simulink model "controller_v12"  (R2022a)
settings: Solver=FixedStepDiscrete  StartTime=0.0  StopTime=inf  RelTol=1e-3
undefined symbols (not defined in the file): ctr, DiscIntNeverNeededParam, flt, IO397, mdl, rbt, rsim, som, ukf_P0_flat, ukf_prediction_time, ukf_s0, ukf_sys, ukf_use_prediction
libraries: simulink x31, slrealtimeloglib x14, slrealtimetgmanagement x5, slrealtimeseriallib x5, speedgoatlib_fpga_analog_io x4, speedgoatlib_fpga x2, speedgoatlib_fpga_dio x1, slrealtimeutilitieslib x1
(part 3 of 4)

== system controller_v12/Adaptive Controller/observer/observer/UKF ==
  r_in : Inport
  euler : Inport  Port=2
  r_dot_in : Inport  Port=3
  omega_in : Inport  Port=4
  f_cmd : Inport  Port=5
  tau_cmd_x : Inport  Port=6
  tau_cmd_y : Inport  Port=7
  To Workspace1 : ToWorkspace  VariableName=ukf_z_in  SaveFormat=Timeseries  SampleTime=-1
  To Workspace2 : ToWorkspace  VariableName=ukf_s  SaveFormat=Timeseries  SampleTime=-1
  To Workspace3 : ToWorkspace  VariableName=ukf_f_cmd  SaveFormat=Timeseries  SampleTime=-1
  To Workspace4 : ToWorkspace  VariableName=ukf_tau_cmd_x  SaveFormat=Timeseries  SampleTime=-1
  To Workspace5 : ToWorkspace  VariableName=ukf_tau_cmd_y  SaveFormat=Timeseries  SampleTime=-1
  UKF_inner : Subsystem
  euler to quat : MATLAB Function  TreatAsAtomicUnit=on
  pack measurement vector : MATLAB Function  TreatAsAtomicUnit=on
  quaternion to rotation matrix : MATLAB Function  TreatAsAtomicUnit=on
  unpack state vector : MATLAB Function  TreatAsAtomicUnit=on
  r_out : Outport
  r_dot_out : Outport  Port=2
  R_out : Outport  Port=3
  omega_out : Outport  Port=4
  wires:
  r_in/1 -> pack measurement vector/1(r)
  r_dot_in/1 -> pack measurement vector/3(r_dot)
  omega_in/1 -> pack measurement vector/4(omega)
  f_cmd/1 -> UKF_inner/2(f_cmd), To Workspace3/1
  tau_cmd_x/1 -> UKF_inner/3(tau_cmd_x), To Workspace4/1
  tau_cmd_y/1 -> To Workspace5/1, UKF_inner/4(tau_cmd_y)
  euler to quat/1(q) -> pack measurement vector/2(q)
  quaternion to rotation matrix/1(R_flat) -> R_out/1
  euler/1 -> euler to quat/1(euler_angles)
  pack measurement vector/1(z_raw) -> UKF_inner/1(z_raw), To Workspace1/1
  unpack state vector/1(r) -> r_out/1
  unpack state vector/2(q) -> quaternion to rotation matrix/1(q)
  unpack state vector/3(r_dot) -> r_dot_out/1
  unpack state vector/4(omega) -> omega_out/1
  UKF_inner/1(s_out) -> unpack state vector/1(s), To Workspace2/1

== system controller_v12/Adaptive Controller/observer/observer/UKF1 ==
  r_in : Inport
  R_in : Inport  Port=2
  f_cmd : Inport  Port=3
  tau_cmd_x : Inport  Port=4
  tau_cmd_y : Inport  Port=5
  s_prediciton_time : Inport  Port=6
  R_flat to quat : MATLAB Function  TreatAsAtomicUnit=on
  Switch : Switch  Criteria=u2 > Threshold  SaturateOnIntegerOverflow=off  InputSameDT=off
  To Workspace1 : ToWorkspace  VariableName=ukf_z_in  SaveFormat=Timeseries  SampleTime=-1
  To Workspace14 : ToWorkspace  VariableName=ukf_s_prediction_out  SaveFormat=Timeseries  SampleTime=-1
  To Workspace2 : ToWorkspace  VariableName=ukf_s  SaveFormat=Timeseries  SampleTime=-1
  To Workspace3 : ToWorkspace  VariableName=ukf_f_cmd  SaveFormat=Timeseries  SampleTime=-1
  To Workspace4 : ToWorkspace  VariableName=ukf_tau_cmd_x  SaveFormat=Timeseries  SampleTime=-1
  To Workspace5 : ToWorkspace  VariableName=ukf_tau_cmd_y  SaveFormat=Timeseries  SampleTime=-1
  UKF_inner : Subsystem
  pack measurement vector : MATLAB Function  TreatAsAtomicUnit=on
  quaternion to rotation matrix : MATLAB Function  TreatAsAtomicUnit=on
  unpack state : MATLAB Function  TreatAsAtomicUnit=on
  use prediction : Constant  Value=ukf_use_prediction
  r_out : Outport
  r_dot_out : Outport  Port=2
  R_out : Outport  Port=3
  omega_out : Outport  Port=4
  wires:
  r_in/1 -> pack measurement vector/1(r)
  f_cmd/1 -> To Workspace3/1, UKF_inner/2(f_cmd)
  tau_cmd_x/1 -> To Workspace4/1, UKF_inner/3(tau_cmd_x)
  tau_cmd_y/1 -> To Workspace5/1, UKF_inner/4(tau_cmd_y)
  R_flat to quat/1(q) -> pack measurement vector/2(q)
  quaternion to rotation matrix/1(R_flat) -> R_out/1
  pack measurement vector/1(z_raw) -> To Workspace1/1, UKF_inner/1(z_raw)
  unpack state/1(r) -> r_out/1
  unpack state/2(q) -> quaternion to rotation matrix/1(q)
  unpack state/3(r_dot) -> r_dot_out/1
  unpack state/4(omega) -> omega_out/1
  R_in/1 -> R_flat to quat/1(R_flat)
  s_prediciton_time/1 -> UKF_inner/5(s_prediction_time)
  Switch/1 -> unpack state/1(s)
  use prediction/1 -> Switch/2
  UKF_inner/2(s_out) -> To Workspace2/1, Switch/3
  UKF_inner/1(s_prediction_out) -> To Workspace14/1, Switch/1

== system controller_v12/Adaptive Controller/observer/observer/lateral observer ==
  XYZ : Inport
  derivative filter : simulink/Discrete/Transfer Fcn Lead or Lag  PoleZ=mdl.zf1  ZeroZ=1  ICPrevOutput=0.0  ICPrevInput=0.0  DoSatur=off
      settings: SourceProductBaseCode=SL
  derivative filter1 : simulink/Discrete/Transfer Fcn Lead or Lag  PoleZ=mdl.zf2  ZeroZ=1  ICPrevOutput=0.0  ICPrevInput=0.0  DoSatur=off
      settings: SourceProductBaseCode=SL
  derivative filter2 : simulink/Discrete/Transfer Fcn Lead or Lag  PoleZ=mdl.zf2  ZeroZ=1  ICPrevOutput=0.0  ICPrevInput=0.0  DoSatur=off
      settings: SourceProductBaseCode=SL
  lat_s : Gain  Gain=mdl.f1
  lat_s2 : Gain  Gain=mdl.f2
  lat_s2_ : Gain  Gain=mdl.f2
  saturation : Subsystem
  r : Outport
  r_dot : Outport  Port=2
  r_dotdot : Outport  Port=3
  wires:
  derivative filter1/1 -> derivative filter2/1
  derivative filter/1 -> lat_s/1
  XYZ/1 -> derivative filter/1, derivative filter1/1, r/1
  derivative filter2/1 -> lat_s2/1
  lat_s/1 -> r_dot/1
  lat_s2/1 -> lat_s2_/1
  lat_s2_/1 -> saturation/1(In1)
  saturation/1(Out1) -> r_dotdot/1

== system controller_v12/Adaptive Controller/observer/ICRA'23/Rotaion/filtered derivative ==
  In1 : Inport
  att_s : Gain  Gain=mdl.f1
  filtered derivative : simulink/Discrete/Transfer Fcn Lead or Lag  PoleZ=mdl.zf1  ZeroZ=1  ICPrevOutput=0.0  ICPrevInput=0.0  DoSatur=off
      settings: SourceProductBaseCode=SL
  low pass3 : DiscreteTransferFcn  Numerator=mdl.vlp.n  Denominator=mdl.vlp.d
  Out1 : Outport
  wires:
  filtered derivative/1 -> low pass3/1
  att_s/1 -> filtered derivative/1
  In1/1 -> att_s/1
  low pass3/1 -> Out1/1

== system controller_v12/Adaptive Controller/observer/ICRA'23/lateral observer/saturation ==
  In1 : Inport
  MinMax2 : MinMax  Inputs=2
  MinMax3 : MinMax  Function=max  Inputs=2
  lw1 : Constant  Value=-mdl.fd_lim
  up1 : Constant  Value=mdl.fd_lim
  Out1 : Outport
  wires:
  In1/1 -> MinMax2/2
  up1/1 -> MinMax2/1
  lw1/1 -> MinMax3/1
  MinMax2/1 -> MinMax3/2
  MinMax3/1 -> Out1/1

== system controller_v12/Adaptive Controller/observer/observer/UKF/UKF_inner ==
  z_raw : Inport
  f_cmd : Inport  Port=2
  tau_cmd_x : Inport  Port=3
  tau_cmd_y : Inport  Port=4
  Delay : Delay  DelayLength=1  InitialCondition="reshape((   diag(vertcat(   1e-4 * ones(12,1),   [0.107 * 7.2e-4; 0.107 * 7.2e-4; 0.107 * 7.2e-4],   [1.1e-21; 1.1e-21; 1e-21]   ))   )',   1,   []   )'"  SampleTime=mdl.T
  Delay1 : Delay  DelayLength=1  InitialCondition=vertcat( [0;0;0], [1;0;0;0], [0;0;0], [0;0;0], [0.981 * 7.2e-4; 0.981 * 7.2e-4; 0.981 * 7.2e-4], [5e-6;5e-6;0] )  SampleTime=mdl.T
  Delay2 : Delay  DelayLength=1  InitialCondition=zeros(13,1)  SampleTime=mdl.T
  Delay3 : Delay  DelayLength=1  InitialCondition=0  SampleTime=mdl.T
  To Workspace3 : ToWorkspace  VariableName=ukf_P_flats  SaveFormat=Timeseries  SampleTime=-1
  UKF update then predict : MATLAB Function  TreatAsAtomicUnit=on  mask{sys=ukf_sys}
  s_out : Outport
  wires:
  z_raw/1 -> UKF update then predict/1(z_raw), Delay2/1
  f_cmd/1 -> UKF update then predict/3(f_cmd)
  tau_cmd_x/1 -> UKF update then predict/4(tau_cmd_x)
  tau_cmd_y/1 -> UKF update then predict/5(tau_cmd_y)
  UKF update then predict/1(s_out) -> s_out/1, Delay1/1
  UKF update then predict/2(P_out_flat) -> Delay/1
  Delay/1 -> UKF update then predict/7(P_in_flat), To Workspace3/1
  Delay1/1 -> UKF update then predict/6(s_in)
  Delay2/1 -> UKF update then predict/2(z_raw_prev)
  UKF update then predict/3(is_init_out) -> Delay3/1
  Delay3/1 -> UKF update then predict/8(is_init_in)

== system controller_v12/Adaptive Controller/observer/observer/UKF1/UKF_inner ==
  z_raw : Inport
  f_cmd : Inport  Port=2
  tau_cmd_x : Inport  Port=3
  tau_cmd_y : Inport  Port=4
  s_prediction_time : Inport  Port=5
  Delay : Delay  DelayLength=1  InitialCondition=ukf_P0_flat  SampleTime=mdl.T
  Delay1 : Delay  DelayLength=1  InitialCondition=ukf_s0  SampleTime=mdl.T
  Delay2 : Delay  DelayLength=1  InitialCondition=[0,0,0, 1,0,0,0,0, 0,0,0, 0,0]'  SampleTime=mdl.T
  Delay3 : Delay  DelayLength=1  InitialCondition=0  SampleTime=mdl.T
  Terminator : Terminator
  To Workspace3 : ToWorkspace  VariableName=ukf_P_flats  SaveFormat=Timeseries  SampleTime=-1
  UKF update then predict : MATLAB Function  TreatAsAtomicUnit=on  mask{sys=ukf_sys}
  bee cov to SI cov : MATLAB Function  TreatAsAtomicUnit=on
  bee units to SI : MATLAB Function  TreatAsAtomicUnit=on
  bee units to SI1 : MATLAB Function  TreatAsAtomicUnit=on
  s_prediction_out : Outport
  s_out : Outport  Port=2
  wires:
  z_raw/1 -> Delay2/1, UKF update then predict/1(z_raw)
  f_cmd/1 -> UKF update then predict/3(f_cmd)
  tau_cmd_x/1 -> UKF update then predict/4(tau_cmd_x)
  tau_cmd_y/1 -> UKF update then predict/5(tau_cmd_y)
  UKF update then predict/1(s_out) -> Delay1/1, bee units to SI/1(s_bee)
  UKF update then predict/2(P_out_flat) -> Delay/1
  Delay/1 -> UKF update then predict/7(P_in_flat), bee cov to SI cov/1(P_flat_bee)
  Delay1/1 -> UKF update then predict/6(s_in)
  Delay2/1 -> UKF update then predict/2(z_raw_prev)
  UKF update then predict/3(is_init_out) -> Delay3/1
  Delay3/1 -> UKF update then predict/8(is_init_in)
  UKF update then predict/4(s_out_pre) -> Terminator/1
  bee units to SI/1(s_si) -> s_out/1
  bee cov to SI cov/1(P_flat_si) -> To Workspace3/1
  UKF update then predict/5(s_prediction_out) -> bee units to SI1/1(s_bee)
  s_prediction_time/1 -> UKF update then predict/9(s_prediction_time)
  bee units to SI1/1(s_si) -> s_prediction_out/1

== system controller_v12/Adaptive Controller/observer/observer/lateral observer/saturation ==
  In1 : Inport
  MinMax2 : MinMax  Inputs=2
  MinMax3 : MinMax  Function=max  Inputs=2
  lw1 : Constant  Value=-mdl.fd_lim
  up1 : Constant  Value=mdl.fd_lim
  Out1 : Outport
  wires:
  In1/1 -> MinMax2/2
  up1/1 -> MinMax2/1
  lw1/1 -> MinMax3/1
  MinMax2/1 -> MinMax3/2
  MinMax3/1 -> Out1/1

== matlab function controller_v12/Adaptive Controller/adaptive setpoint rd ==
  data: rd output; rd_d output; rd_dd output; rd_ddd output; rd_dddd output; time input; r input; r_d input; landing input; som_ph input; ctr parameter; som parameter; mdl parameter
function [rd,rd_d,rd_dd,rd_ddd,rd_dddd] = fcn(time, r, r_d, landing,som_ph, ctr, som, mdl)
%#codegen

rd = [ctr.setpoint.x; ctr.setpoint.y; ctr.setpoint.z];
rd_d = zeros(3,1);
rd_dd = zeros(3,1);
rd_ddd = zeros(3,1);
rd_dddd = zeros(3,1);

if time <= mdl.i_delay
    rd_z = 0;
    rd   = [ctr.setpoint.x; ctr.setpoint.y; rd_z];
end

% takeoff
if ctr.takeoff.en
    if time > mdl.i_delay && time < (mdl.i_delay+ctr.takeoff.time)
        rd_z = ctr.takeoff.height + (((ctr.setpoint.z-ctr.takeoff.height)/ctr.takeoff.time)*(time-mdl.i_delay));
        if rd_z > ctr.setpoint.z
            rd_z = ctr.setpoint.z;
        end
        rd   = [ctr.setpoint.x; ctr.setpoint.y; rd_z];
    end
end

% planned landing 
if ctr.landing.en
    if time > (mdl.rt-ctr.landing.time)
        rd_z = ctr.setpoint.z-(((ctr.setpoint.z-ctr.landing.height)/ctr.landing.time)*(time-mdl.rt+ctr.landing.time));
        if rd_z < ctr.landing.height
            rd_z = ctr.landing.height;
        end
        rd   = [ctr.setpoint.x; ctr.setpoint.y; rd_z];
    end
end

% forced landing
if landing
    rd_z = 0.02;
    rd   = [ctr.setpoint.x; ctr.setpoint.y; rd_z];
end


% somersault
if som.en
    if time > som.t_start + som.t_rise + som.t_acc + som.t_dcc + som.t_rec
        % % afterwards 
        %dt = som.t_start + som.t_rise + som.t_acc + som.t_dcc + som.t_rec - time;
        %rd = rd + dt*(r-rd);
    elseif time > som.t_start + som.t_rise + som.t_acc + som.t_dcc
        % recovery
        dt = som.t_start + som.t_rise + som.t_acc + som.t_dcc + som.t_rec - time;
        rd = rd + (dt/som.t_rec)*(r-rd);
        rd_d = rd_d + 0.5*(dt/som.t_rec)*(r_d-rd_d);
        rd(1) = min(max(rd(1),-0.25),0.25); % 25 cm envelope
        rd(2) = min(max(rd(2),-0.25),0.25); % 25 cm envelope
        rd(3) = max(rd(3),0.02); % min altitude setpoint.
    end
end


end

== matlab function controller_v12/Force//Torque to Trajectory Specs/nominal desired voltage/force to voltage (hovering) /MATLAB Function ==
  data: Vi input; Vo output; mdl parameter
function Vo = fcn(Vi,mdl)
%old script
% if max(Vi)>mdl.max_v
%     Vo = Vi * mdl.max_v/max(Vi);
%     % scale down all votages if one exceeds the max limit.
% else
%     Vo = Vi;
% end

%new change (modify max_v to a vector so each DEA has its own max)
% scale_down_ratio_vec = Vi ./ mdl.max_v_vec;
% scale_down_ratio = max(scale_down_ratio_vec);
% bool_scale_down = scale_down_ratio>1;
% 
% if bool_scale_down
%    Vo = Vi/scale_down_ratio;
% else
%    Vo = Vi; 
% end

min_v_vec = mdl.hovering_vec -150;
scale_down_ratio_vec = (Vi-min_v_vec)./(mdl.max_v_vec-min_v_vec);

scale_down_ratio = max(scale_down_ratio_vec);
bool_scale_down = scale_down_ratio>1;

if bool_scale_down
    Vo = min_v_vec + (Vi - min_v_vec)./scale_down_ratio;	
else
	  Vo = Vi; 
end


%extra layer of safety
for i=1:length(Vo)
	Vo(i) = min(Vo(i),mdl.max_v_vec(i));
end

== matlab function controller_v12/Adaptive Controller/somersault_phase ==
  data: som_phase output; time input; mdl parameter; som parameter
function som_phase  = fcn(time, mdl, som)
%#codegen

som_phase = 0;  % during a normal flight
if som.en
    if time > som.t_start + som.t_rise + som.t_acc + som.t_dcc + som.t_rec
        som_phase = 0;  % afterwards
    elseif time > som.t_start + som.t_rise + som.t_acc + som.t_dcc
        som_phase = 4;  % recovery
    elseif time > som.t_start + som.t_rise + som.t_acc
        som_phase = 3;  % rolling, second half.
    elseif time > som.t_start + som.t_rise
        som_phase = 2;  % rolling, first half.
    elseif time > som.t_start
        som_phase = 1;  % gaining altitude
    end
end

== matlab function controller_v12/Force//Torque to Trajectory Specs/nominal desired voltage/force to voltage flipping/MATLAB Function ==
  data: Vi input; Vo output; mdl parameter
function Vo = fcn(Vi,mdl)
%old script
% if max(Vi)>mdl.max_v
%     Vo = Vi * mdl.max_v/max(Vi);
%     % scale down all votages if one exceeds the max limit.
% else
%     Vo = Vi;
% end

%new change (modify max_v to a vector so each DEA has its own max)
scale_down_ratio_vec = Vi ./ mdl.max_v_vec;
scale_down_ratio = max(scale_down_ratio_vec);
bool_scale_down = scale_down_ratio>1;

if bool_scale_down
   Vo = Vi/scale_down_ratio;
else
   Vo = Vi; 
end

== matlab function controller_v12/smothing/smoothing ==
  data: time input; out_amp output; amp input; amp2 input; som parameter
function out_amp  = fcn(time,amp,amp2,som)
%#codegen

alp = 1;
if time > som.t_start + som.t_rise + som.t_acc + som.t_dcc + som.t_rec
    alp = 1;  % afterwards
elseif time > som.t_start
    alp = som.filter.alp;
end
% set en = 0 if the robot goes out of the safe envelope.
out_amp = som.filter.alp*amp + (1-som.filter.alp)*amp2;

== matlab function controller_v12/Adaptive Controller/saturation ==
  data: x_roll input; X_roll output size=1; y_pitch input; z_yaw input; Y_pitch output size=1; Z_yaw output size=1; Th input; Force output size=1; rbt parameter; ctr parameter; som_phase input; som parameter
function [X_roll, Y_pitch, Z_yaw, Force] = fcn(x_roll, y_pitch, z_yaw, Th, rbt, ctr, som_phase, som)
%#codegen

X_roll = max(min(x_roll, ctr.lim.taux), -ctr.lim.taux);
%X_roll = x_roll;
Y_pitch = max(min(y_pitch, ctr.lim.tauy), -ctr.lim.tauy);
%Y_pitch = y_pitch;
Z_yaw = max(min(z_yaw, ctr.lim.tauz), -ctr.lim.tauz);

Force = Th*rbt.m;

% F is already checked for saturation, but still needs to be converted into
% Newton

%% Roll torque management (somersault)
if som_phase == 2
    X_roll = som.roll_mag; % torque in SI
    Y_pitch = 0;  % to turn of the pitch control
elseif som_phase == 3
    X_roll = -som.roll_mag; % torque in SI
    Y_pitch = 0;  % to turn of the pitch control
end
    
%% Thrust management
% thrust is not controlled during the flipping maneuver (the output here will be overridden in the mapping).

== matlab function controller_v12/Force//Torque to Trajectory Specs/force//torque to module thrust/mapping scheme (flipping compataible) ==
  data: time input; module_f output; inputs input; rbt parameter; som parameter; mdl parameter
function module_f  = fcn(time, inputs, rbt, som, mdl)

% somersault
if som.en
    if time > som.t_start + som.t_rise + som.t_acc + som.t_dcc+som.t_rec % after recovery
        %
    elseif time > som.t_start + som.t_rise + som.t_acc + som.t_dcc % recovery
        %inputs(1) = rbt.m*(mdl.g*(som.thrust_f+0.2));
    elseif time > som.t_start + som.t_rise % rolling, first half+second half.
        % priortize the roll torque and ensure non-negative forces.
        inputs(1) = 0;
    elseif time > som.t_start
        inputs(1) = rbt.m*(mdl.g*som.thrust_f); % during the t rise.                
    end
end

% torque/thrust to unit force mapping
if rbt.til == 0
    module_f = rbt.Apinv * inputs(1:3); % original mapping
elseif rbt.til > 0
    module_f = rbt.A2inv * inputs;
else
    module_f = [0 0 0 0]';
end

% safety
if min(module_f) < 0
    module_f = module_f - min(module_f); % this ensure positive module forces
end

end

== matlab function controller_v12/Adaptive Controller/adaptive system/integrator/initial guess ==
  data: i_e input; int_e output; tor_off input; th_off input; tor_inte output; th_inte output; ctr parameter; rbt parameter; mdl parameter
function [int_e, tor_inte, th_inte] = fcn(i_e, tor_off, th_off, ctr, rbt, mdl)
%#codegen

tor_inte = zeros(3,1);
int_e    = zeros(4,1);

int_e(1) = i_e(1)+tor_off(1);
int_e(2) = i_e(2)+tor_off(2);
int_e(3) = i_e(3)+tor_off(3);
int_e(4) = i_e(4)+th_off;

tor_inte(1) = int_e(1)*ctr.gain.ati*rbt.ixx/mdl.g;
tor_inte(2) = int_e(2)*ctr.gain.ati*rbt.iyy/mdl.g;
tor_inte(3) = 0;

th_inte     = int_e(4)*ctr.gain.ali;

== matlab function controller_v12/Phantom trigger/start at one ==
  data: time input; trigger output
function trigger = fcn(time)
%#codegen
trigger = 0;
if time > 1
   trigger = 1; 
end
if time > 2
   trigger = 0; 
end

== matlab function controller_v12/Measurement manager/safety check system/envelope check ==
  data: x input; en output; y input; z input; ctr parameter
function en  = fcn(x,y,z, ctr)

if abs(x)>ctr.safety.enableZone.xmax || abs(y)>ctr.safety.enableZone.ymax || abs(z)>ctr.safety.enableZone.zmax
    en = 0;
else
    en = 1;
end

end

== matlab function controller_v12/Dynamic Sim/conditioning ==
  data: Rout output; Rin input; eu output
function [Rout, eu]  = fcn(Rin)
%#codegen
Rm = [Rin(1:3)./norm(Rin(1:3)),Rin(4:6)./norm(Rin(4:6)),Rin(7:9)./norm(Rin(7:9))];
% conditioning on orthogonality.
Rout = [Rm(:,1);Rm(:,2);Rm(:,3)];

% euler angles
euy = asin(min(max(Rm(1,3),-1),1));
eux = atan2(-Rm(2,3),Rm(3,3));
euz = atan2(-Rm(1,2),Rm(1,1));
%euz=acos(min(max(Rm(1,1)/cos(euy),-1),1));
%eux=acos(min(max(Rm(3,3)/cos(euy),-1),1));
eu = [eux;euy;euz];
% not being very careful with singularities.

== matlab function controller_v12/Force//Torque to Trajectory Specs/nominal desired voltage/map_selection ==
  data: hover_map output; time input; mdl parameter; som parameter
function hover_map  = fcn(time, mdl, som)
%#codegen

hover_map = 1;  % during a normal flight
if som.en
    if time > som.t_start + som.t_rise + som.t_acc + som.t_dcc
        hover_map = 1;  % afterwards
    elseif time > som.t_start + som.t_rise
    %elseif time > som.t_start + som.t_rise 
        hover_map = 0;  % 
    end
end

== matlab function controller_v12/Dynamic Sim/rigid body dynamics sim ==
  data: dv output double size=3; mforces input double; dR output double size=9; dw output double size=3; v input; R input; w input; rbt parameter; mdl parameter; disturbance input; rsim parameter
function [dv, dR, dw]  = fcn(mforces,v,R,w,rbt,mdl,disturbance, rsim)
%#codegen

% noiseless
% no damping
% rbt_A_temp = [rbt.A; 0.015 -0.015 0.015 -0.015];
rbt_A_temp = rbt.A2;
% inputs = rbt.A * mforces(:);
inputs = rbt_A_temp * mforces(:);
thrust = inputs(1);
% torque = [inputs(2);inputs(3);0];
torque = [inputs(2);inputs(3);inputs(4)];
%R = R(:);
%w = w(:);
dv = R(7:9)*thrust/rbt.m - [0;0;mdl.g] + disturbance(1:3);

dw = diag([rsim.rbt.ixx, rsim.rbt.iyy, rsim.rbt.izz]) \ ( (torque) - cross(w,diag([rsim.rbt.ixx, rsim.rbt.iyy, rsim.rbt.izz])*w)+ disturbance(4:6) ) ;
dR1 = R(4:6)*w(3)-R(7:9)*w(2);
dR2 = R(7:9)*w(1)-R(1:3)*w(3);
dR3 = R(1:3)*w(2)-R(4:6)*w(1);
dR = [dR1;dR2;dR3];
%dv = zeros(3,1);
%dw = zeros(3,1);
%dR = zeros(9,1);

== matlab function controller_v12/Adaptive Controller/attitude and thrust MPC controller/External Torque Observer ==
  data: time input; omega input; omega_hat output; torque_x input; torque_y input; ext_torque_hat input; omega_hat input; ext_torque_hat output; ctr parameter; rbt parameter; mdl parameter
function [omega_hat, ext_torque_hat] = fcn(time, omega, torque_x, torque_y, ext_torque_hat, omega_hat, ctr, rbt, mdl)
   
if time > mdl.i_delay
     
    omega_hat = omega_hat(:);
    ext_torque_hat = ext_torque_hat(:);
    J = diag([rbt.ixx, rbt.iyy, rbt.izz]);
    omega_cross_J_omega = cross(omega, J*omega);
    x_hat_curr = diag(ctr.torque_obs.state_scaling)*[omega_hat(:); ext_torque_hat(:)];
    u = diag(ctr.torque_obs.input_scaling)*[torque_x - omega_cross_J_omega(1); torque_y - omega_cross_J_omega(2)];
    y = diag(ctr.torque_obs.meas_scaling)*omega(1:2); 
    x_hat_pred = ctr.torque_obs.A*x_hat_curr + ctr.torque_obs.B(:, 1:2)*u; 
    x_hat_next = diag(ctr.torque_obs.out_scaling)*(x_hat_pred + ctr.torque_obs.L*(y - ctr.torque_obs.C*x_hat_pred));
    omega_hat = x_hat_next(1:2,1);
    ext_torque_hat = x_hat_next(3:4,1);
end

end

== matlab function controller_v12/Measurement manager/safety check system/voltage check ==
  data: voltage input; en output; ctr parameter
function en  = fcn(voltage, ctr)

if sum(voltage>ctr.safety.volt) > 0
    en = 0;
else
    en = 1;
end

end

== matlab function controller_v12/Measurement manager/envelope//voltage check ==
  data: x input; keep_flying output size=1; y input; z input; ctr parameter
function keep_flying  = fcn(x,y,z,ctr)

if abs(x)>ctr.safety.land.xmax || abs(y)>ctr.safety.land.ymax || abs(z)>ctr.safety.land.zmax
    keep_flying = 0;
% elseif voltage(1) > ctr.safety.land.volt
%     keep_flying = 0;    
else
    keep_flying = 1;
end

end

== matlab function controller_v12/Measurement manager/MATLAB Function ==
  data: keep_flying input; landing_in input; landing_out output size=1; cum_in input; cum_out output size=1; ctr parameter; mdl parameter
function [landing_out, cum_out] = fcn(keep_flying, landing_in, cum_in, ctr, mdl)

if keep_flying == 0
    cum_out = cum_in + mdl.T;
else
    cum_out = 0;
end

if cum_out > ctr.safety.land.T || landing_in == 1
    landing_out = 1;
else 
    landing_out = 0;
end

end

== matlab function controller_v12/Measurement manager/voltage check ==
  data: voltage input; keep_flying output size=1; ctr parameter
function keep_flying  = fcn(voltage, ctr)

% if voltage(1)>ctr.safety.land.volt || voltage(2)>ctr.safety.land.volt || voltage(3)>ctr.safety.land.volt || voltage(4)>ctr.safety.land.volt

if sum(voltage>ctr.safety.land.volt)>0
    keep_flying = 0;
else
    keep_flying = 1;
end

end

== matlab function controller_v12/Measurement manager/safety check system/MATLAB Function ==
  data: keep_flying input; en_in input; en_out output size=1; cum_in input; cum_out output size=1; ctr parameter; mdl parameter
function [en_out, cum_out] = fcn(keep_flying, en_in, cum_in, ctr, mdl)

if keep_flying == 0
    cum_out = cum_in + mdl.T;
else
    cum_out = 0;
end

if cum_out > ctr.safety.T || en_in == 0
    en_out = 0;
else 
    en_out = 1;
end

end

== matlab function controller_v12/MATLAB Function ==
  data: u input; y output
function y = fcn(u)

y = u;

== matlab function controller_v12/Adaptive Controller/attitude and thrust MPC controller/PD Atttiude Controller ==
  data: time input; cmd_B_torque output; R input; Omega input; Rd input; Omegad input; tau_ext input; ctr parameter; rbt parameter; mdl parameter; att_e output
function [cmd_B_torque, att_e]   = fcn(time, R, Omega, Rd, Omegad, tau_ext, ctr, rbt, mdl)
%#codegen
% r: curr pos
% r_dot: curr vel
% R: current attitude
% Omega: current body rates
% rd : des pos
% rd_d: des vel
% Rd: desired attitude (rotation matrix)
% Omegad: desired angular velocity


% current attitude
R = get_rotation_matrix(R);     % transform vector in rotation matrix
Omega = Omega(:);
Omegad = Omegad(:);

% desired attitude & angvel
Rd = get_rotation_matrix(Rd);

B_ypr_curr = rotm2eul(R);
B_ypr_des = rotm2eul(Rd);

B_ypr_dot_des = get_euler_derivatives(B_ypr_des, Omegad);
B_ypr_dot_curr = get_euler_derivatives(B_ypr_curr, Omega);
B_ypr_e_dot = (B_ypr_dot_curr - B_ypr_dot_des);
B_rpy_e_dot = [B_ypr_e_dot(3); B_ypr_e_dot(2); B_ypr_e_dot(1)];
disp(B_rpy_e_dot)
disp(Omega - Omegad)

B_ypr_e = B_ypr_curr - B_ypr_des;
B_rpy_e = [B_ypr_e(3); B_ypr_e(2); B_ypr_e(1)];
M = diag(ctr.att_pid_e)*B_rpy_e + diag(ctr.att_pid_e_dot)*B_rpy_e_dot + [tau_ext(1); tau_ext(2); 0.0];

%att_e = eR'*eR; % squared norm of the error
att_e = B_rpy_e(:);
cmd_B_torque = M(:);
end

function R = get_rotation_matrix(R)
    R11 = R(1);
    R12 = R(2);
    R13 = R(3);
    R21 = R(4);
    R22 = R(5);
    R23 = R(6);
    R31 = R(7);
    R32 = R(8);
    R33 = R(9);
    R1 = [R11; R21; R31];     % unit (column) vector
    R2 = [R12; R22; R32];
    R3 = [R13; R23; R33];
    R = [R1, R2, R3];
end

function [B_ypr_dot] = get_euler_derivatives(B_ypr, B_omega)
% https://www.astro.rug.nl/software/kapteyn-beta/_downloads/attitude.pdf
sy = sin(B_ypr(1));
cy = cos(B_ypr(1));
sp = sin(B_ypr(2));
cp = cos(B_ypr(2));
E_zyx = [[0; 0; 1], [-sy; cy; 0.0], [cy*cp; sy*cp; -sp]];
B_ypr_dot = E_zyx\B_omega;

end

== matlab function controller_v12/Adaptive Controller/attitude and thrust MPC controller/Pakpong;s atttiude ==
  data: time input; R input; Omega input; Rd input; Omegad input; cmd_B_acc_z input; cmd_B_torque output; ctr parameter; rbt parameter; mdl parameter; att_e output
function [cmd_B_torque, att_e]   = fcn(time, R, Omega, Rd, Omegad, cmd_B_acc_z, ctr, rbt, mdl)
%#codegen

%% init
R11 = R(1);
R12 = R(2);
R13 = R(3);
R21 = R(4);
R22 = R(5);
R23 = R(6);
R31 = R(7);
R32 = R(8);
R33 = R(9);
R1 = [R11; R21; R31];     % unit (column) vector
R2 = [R12; R22; R32];
R3 = [R13; R23; R33];
R = [R1, R2, R3];
wx = Omega(1);
wy = Omega(2);
wz = Omega(3);

e3 = [0; 0; 1];
rd_dd = get_rotation_matrix(Rd)*e3*cmd_B_acc_z;

torque_x = ...
- ctr.gain.at3*( mdl.g*wx) - ...
ctr.gain.at2*( dot(R2,rd_dd) );
torque_x = torque_x*rbt.ixx/mdl.g;

torque_y = ...
- ctr.gain.at3*( mdl.g*wy) - ...
ctr.gain.at2*( dot(R1,-rd_dd) );
torque_y = torque_y*rbt.iyy/mdl.g;

torque_z = 0;           % no yaw control

att_e = -[-dot(R2,rd_dd);dot(R1,rd_dd);0];

cmd_B_torque = [torque_x; torque_y; torque_z];

end

function R = get_rotation_matrix(R)
    R11 = R(1);
    R12 = R(2);
    R13 = R(3);
    R21 = R(4);
    R22 = R(5);
    R23 = R(6);
    R31 = R(7);
    R32 = R(8);
    R33 = R(9);
    R1 = [R11; R21; R31];     % unit (column) vector
    R2 = [R12; R22; R32];
    R3 = [R13; R23; R33];
    R = [R1, R2, R3];

end

== matlab function controller_v12/Adaptive Controller/attitude and thrust MPC controller2/Geometric Attitude Controller ==
  data: time input; torque_x output; R input; Omega input; Rd input; Omegad input; ctr parameter; rbt parameter; torque_y output; torque_z output; mdl parameter; att_e output
function [torque_x, torque_y, torque_z, att_e]   = fcn(time, R, Omega, Rd, Omegad, ctr, rbt, mdl)
%#codegen
% r: curr pos
% r_dot: curr vel
% R: current attitude
% Omega: current body rates
% rd : des pos
% rd_d: des vel
% Rd: desired attitude (rotation matrix)
% Omegad: desired angular velocity


% current attitude
R = get_rotation_matrix(R);     % transform vector in rotation matrix
Omega = Omega(:);

% desired attitude & angvel
Rd = get_rotation_matrix(Rd);
Omegad = Omegad(:);
% Omegad      = [0; 0; 0]; % vee(Rd.'*Rd_1dot);
Omegad_1dot = [0; 0; 0]; % vee(Rd.'*Rd_2dot - hat(Omegad)*hat(Omegad));

% inertia matrix
J = diag([ctr.lee.ixx, ctr.lee.iyy, ctr.lee.izz]);

% attitude and angular velocity errors
eR     = (1/2)*vee(Rd.'*R - R.'*Rd);
eOmega = Omega - R.'*Rd*Omegad;

% desired torque
M = -ctr.lee.kR*eR - ctr.lee.kOmega*eOmega + cross(Omega, J*Omega) ...
  - J*(hat(Omega)*R.'*Rd*Omegad - R.'*Rd*Omegad_1dot);

%att_e = eR'*eR; % squared norm of the error
att_e = eR;

torque_x = M(1);
torque_y = M(2);
torque_z = M(3);

end

function vec = vee(ss)
% function vec = vee(skewsymmetric)
%   The vee function maps a skew-symmetric 
%   matrix to a vector

% https://github.com/justinthomas/MATLAB-tools/blob/master/vee.m

if isa(ss,'sym')
    ss = expand(simplify(ss));
end

switch numel(ss)
    
    case 4
        
        if ~isequal(ss(1,2), -ss(2,1))
            %warning('The provided matrix is not skew symmetric')
        end
        
        vec = ss(1,2);

    case 9

        if ~isequal(ss(3,2),-ss(2,3)) || ~isequal(ss(1,3),-ss(3,1)) || ~isequal(ss(2,1),-ss(1,2))
            %warning('The provided matrix is not skew symmetric.')
            %print(ss)
        end

        vec = [ss(3,2); ss(1,3); ss(2,1)];
end

if isa(ss,'sym')
    vec = simplify(vec);
end

end

function ss = hat(vec)
% function ss = hat(vec)
%   The hat function maps a vector in R^3 (or R^1) to its
%   skew symmetric matrix in R^(3x3) (or R^(2x2))

% https://github.com/justinthomas/MATLAB-tools/blob/master/hat.m

switch length(vec)
    
    case 3
        ss = [...
            0, -vec(3), vec(2);...
            vec(3), 0, -vec(1);...
            -vec(2), vec(1), 0];
        
    case 1
        ss = [...
            0, vec; ...
            -vec, 0];
end

end

function R = get_rotation_matrix(R)
    R11 = R(1);
    R12 = R(2);
    R13 = R(3);
    R21 = R(4);
    R22 = R(5);
    R23 = R(6);
    R31 = R(7);
    R32 = R(8);
    R33 = R(9);
    R1 = [R11; R21; R31];     % unit (column) vector
    R2 = [R12; R22; R32];
    R3 = [R13; R23; R33];
    R = [R1, R2, R3];

end

== matlab function controller_v12/Adaptive Controller/attitude and thrust MPC controller2/MATLAB Function ==
  data: u input; y output
function y = fcn(u)

y = u;

== matlab function controller_v12/Adaptive Controller/attitude and thrust MPC controller/Geometric Attitude Controller ==
  data: time input; cmd_B_torque output; R input; Omega input; Rd input; Omegad input; tau_ext input; ctr parameter; rbt parameter; mdl parameter; att_e output
function [cmd_B_torque, att_e]   = fcn(time, R, Omega, Rd, Omegad, tau_ext, ctr, rbt, mdl)
%#codegen
% r: curr pos
% r_dot: curr vel
% R: current attitude
% Omega: current body rates
% rd : des pos
% rd_d: des vel
% Rd: desired attitude (rotation matrix)
% Omegad: desired angular velocity


% current attitude
R = get_rotation_matrix(R);     % transform vector in rotation matrix
Omega = Omega(:);
Omegad = Omegad(:);

% desired attitude & angvel
Rd = get_rotation_matrix(Rd);
% inertial frame 3-axis



% thrust magnitude control, eq 19
%A = -ctr.lee.pos.kx*ex - ctr.lee.pos.kv*ev - rbt.m*mdl.g*e3; % + P.mass*xd_2dot;
%cmd_B_acc_z = dot(-A, R*e3)/rbt.m;

Rd = get_desired_attitude_x_axis(Rd, R);
%Rd = get_desired_attitude_y_axis(Rd, R);

% inertia matrix
J = diag([ctr.lee.ixx, ctr.lee.iyy, ctr.lee.izz]);

% attitude and angular velocity errors
eR     = (1/2)*vee(Rd.'*R - R.'*Rd);
eOmega = Omega - R.'*Rd*Omegad;
% desired torque
M = -ctr.lee.kR*eR - ctr.lee.kOmega*eOmega + cross(Omega, J*Omega)...
    - J*(hat(Omega)*R.'*Rd*Omegad) ...
    - ctr.torque_obs.factor.*[tau_ext(1); tau_ext(2); 0.0]; % ...
  % - J*(- R.'*Rd*Omegad_1dot);
  % - J*(hat(Omega)*R.'*Rd*Omegad) ...

%att_e = eR'*eR; % squared norm of the error
att_e = eR;
cmd_B_torque = M(:);
end

function vec = vee(ss)
% function vec = vee(skewsymmetric)
%   The vee function maps a skew-symmetric 
%   matrix to a vector

% https://github.com/justinthomas/MATLAB-tools/blob/master/vee.m

if isa(ss,'sym')
    ss = expand(simplify(ss));
end

switch numel(ss)
    
    case 4
        
        if ~isequal(ss(1,2), -ss(2,1))
            disp('The provided matrix is not skew symmetric')
        end
        
        vec = ss(1,2);

    case 9

        if ~isequal(ss(3,2),-ss(2,3)) || ~isequal(ss(1,3),-ss(3,1)) || ~isequal(ss(2,1),-ss(1,2))
            disp('The provided matrix is not skew symmetric.')
            %print(ss)
        end

        vec = [ss(3,2); ss(1,3); ss(2,1)];
end

if isa(ss,'sym')
    vec = simplify(vec);
end

end

function ss = hat(vec)
% function ss = hat(vec)
%   The hat function maps a vector in R^3 (or R^1) to its
%   skew symmetric matrix in R^(3x3) (or R^(2x2))

% https://github.com/justinthomas/MATLAB-tools/blob/master/hat.m

switch length(vec)
    
    case 3
        ss = [...
            0, -vec(3), vec(2);...
            vec(3), 0, -vec(1);...
            -vec(2), vec(1), 0];
        
    case 1
        ss = [...
            0, vec; ...
            -vec, 0];
end

end

function R = get_rotation_matrix(R)
    R11 = R(1);
    R12 = R(2);
    R13 = R(3);
    R21 = R(4);
    R22 = R(5);
    R23 = R(6);
    R31 = R(7);
    R32 = R(8);
    R33 = R(9);
    R1 = [R11; R21; R31];     % unit (column) vector
    R2 = [R12; R22; R32];
    R3 = [R13; R23; R33];
    R = [R1, R2, R3];

end

function Omegad = get_desired_body_velocity()

% time derivatives of body axes -- arXiv:1003.2005v3, Appendix F
A_1dot   = -ctr.lee.pos.kx*ev; %- ctr.lee.pos.kv*ea + ctr.lee.pos.mass*xd_3dot;
b3c_1dot = -A_1dot/norm(A) + (dot(A,A_1dot)/norm(A)^3)*A;
C_1dot   = cross(b3c_1dot, b1d) + cross(b3c, b1d_1dot);
b2c_1dot = C/norm(C) - (dot(C,C_1dot)/norm(C)^3)*C;
% b2c_1dot = -1*b2c_1dot;
b1c_1dot = cross(b2c_1dot, b3c) + cross(b2c, b3c_1dot);

% Extract calculated angular velocities and their time-derivatives
Rd_1dot     = [b1c_1dot b2c_1dot b3c_1dot];
Omegad      = vee(Rd_tmp.'*Rd_1dot);

% Omegad      = [0; 0; 0]; % vee(Rd.'*Rd_1dot);
Omegad_1dot = [0; 0; 0]; % vee(Rd.'*Rd_2dot - hat(Omegad)*hat(Omegad));

end

function Rd = get_desired_attitude_x_axis(Rd, R)

    e3 = [0;0;1];
    % normalized feedback function, eq 23
    b3c = Rd*e3;
    
    % Desired x axis -- current x axis
    b1d = R(:, 1);
    
    % Construct b1c, eq 38
    C = cross(b3c, b1d); % arXiv:1003.2005v3, eq ~97
    b1c = -(1/norm(C))*cross(b3c, C);
    
    b2c = C/norm(C);
    
    % computed attitude, eq 22
    Rd = [b1c b2c b3c];

end


function Rd = get_desired_attitude_y_axis(Rd, R)

    e3 = [0;0;1];
    % normalized feedback function, eq 23
    b3c = Rd*e3;
    
    % Desired y axis -- current x axis
    b2d = R(:, 2);
    
    % Construct b2c, eq 38
    C = cross(b3c, b2d); % arXiv:1003.2005v3, eq ~97
    b2c = -(1/norm(C))*cross(b3c, C);
    
    b1c = C/norm(C);
    
    % computed attitude, eq 22
    Rd = [b1c b2c b3c];

end

== matlab function controller_v12/Adaptive Controller/attitude and thrust MPC controller/Geometric Controller ==
  data: time input; r input; Rd output; r_dot input; r_dotdot input; R input; Omega input; rd input; rd_d input; rd_dd input; rd_ddd input; rd_dddd input; int_e input; ctr parameter; rbt parameter; Omegad output; cmd_B_acc_z output; mdl parameter; alt_e output; rd_rtmpc output
function [Rd, Omegad, cmd_B_acc_z, alt_e, rd_rtmpc]   = fcn(time, r, r_dot, r_dotdot, R, Omega, rd,rd_d,rd_dd,rd_ddd,rd_dddd, int_e, ctr, rbt, mdl)
    %#codegen
    % r: curr pos
    % r_dot: curr vel
    % R: current attitude
    % Omega: current body rates
    % rd : des pos
    % rd_d: des vel
    %% Out: 
    % cmd_B_thrust_z is thrust force on z axis in body (B) frame [N]
    
    % Ensure signals have expected shape
    R11 = R(1);
    R12 = R(2);
    R13 = R(3);
    R21 = R(4);
    R22 = R(5);
    R23 = R(6);
    R31 = R(7);
    R32 = R(8);
    R33 = R(9);
    R1 = [R11; R21; R31];     % unit (column) vector
    R2 = [R12; R22; R32];
    R3 = [R13; R23; R33];
    R = [R1, R2, R3];

    r = r(:);           % position
    r_dot = r_dot(:);   % velocity 

    rd = rd(:);         % desired position
    rd_d = rd_d(:);     % desired velocity

    rd_rtmpc = [rd; rd_d];

    
    % From https://github.com/plusk01/se3quad/blob/master/matlab/controller.m
    % calculate errors, eq 17-18
    ex = r - rd;
    ev = r_dot - rd_d;
    %ea = v_1dot - xd_2dot;
    %ej = v_2dot - xd_3dot;
    
    % inertial frame 3-axis
    e3 = [0;0;1];
    
    % thrust magnitude control, eq 19
    A = -ctr.lee.pos.kx*ex - ctr.lee.pos.kv*ev - rbt.m*mdl.g*e3; % + P.mass*xd_2dot;
    cmd_B_acc_z = dot(-A, R*e3)/rbt.m;
    
    % normalized feedback function, eq 23
    b3c = -A/norm(A);

    % Desired x axis -- current x axis
    b1d = R(:, 1);
    % Desired angular velocity of this axis - zero?
    b1d_1dot = [0; 0; 0];
    
    % Construct b1c, eq 38
    C = cross(b3c, b1d); % arXiv:1003.2005v3, eq ~97
    b1c = -(1/norm(C))*cross(b3c, C);
    
    b2c = C/norm(C);
    
    % computed attitude, eq 22
    Rd_tmp = [b1c b2c b3c];

    % time derivatives of body axes -- arXiv:1003.2005v3, Appendix F
    A_1dot   = -ctr.lee.pos.kx*ev; %- ctr.lee.pos.kv*ea + ctr.lee.pos.mass*xd_3dot;
    b3c_1dot = -A_1dot/norm(A) + (dot(A,A_1dot)/norm(A)^3)*A;
    C_1dot   = cross(b3c_1dot, b1d) + cross(b3c, b1d_1dot);
    b2c_1dot = C/norm(C) - (dot(C,C_1dot)/norm(C)^3)*C;
    % b2c_1dot = -1*b2c_1dot;
    b1c_1dot = cross(b2c_1dot, b3c) + cross(b2c, b3c_1dot);
    
    % Extract calculated angular velocities and their time-derivatives
    Rd_1dot     = [b1c_1dot b2c_1dot b3c_1dot];
    Omegad      = vee(Rd_tmp.'*Rd_1dot);

    % Desired angular velocity
    % Omegad = [0.0, 0.0, 0.0]; % TODO

    % Altitude error
    alt_e = r(3) - rd(3); 

    % Generate output. 
    Rd_tmp = Rd_tmp'; % this is needed to respect existing convention that rot. matrices are passed
          % around as vectors, created by concatenating the rows of the
          % matrix (and Rd(:) will created a vector by concatentatig the columns of Rd)
    Rd = Rd_tmp(:);
end

function [B_thrust] = compensate_thrust(cmd_B_acc_z, B_ypr, mass, g)
    B_thrust_z = mass * (cmd_B_acc_z+g)/cos(B_ypr(3))/cos(B_ypr(2));
    B_thrust = [0.0; 0.0; B_thrust_z];
end

function [B_roll, B_pitch] = compensate_attitude(B_thrust, lin_B_roll, lin_B_pitch, mass, g)
    B_acc_z = (B_thrust(3))/mass;
    B_roll = lin_B_roll*(g/B_acc_z);
    B_pitch = lin_B_pitch*(g/B_acc_z);
end

function [R] = get_B_R_yaw_I(yaw)
    R = [cos(yaw), sin(yaw); -sin(yaw), cos(yaw)];
end

function vec = vee(ss)
% function vec = vee(skewsymmetric)
%   The vee function maps a skew-symmetric 
%   matrix to a vector

% https://github.com/justinthomas/MATLAB-tools/blob/master/vee.m

if isa(ss,'sym')
    ss = expand(simplify(ss));
end

switch numel(ss)
    
    case 4
        
        if ~isequal(ss(1,2), -ss(2,1))
            %warning('The provided matrix is not skew symmetric')
        end
        
        vec = ss(1,2);

    case 9

        if ~isequal(ss(3,2),-ss(2,3)) || ~isequal(ss(1,3),-ss(3,1)) || ~isequal(ss(2,1),-ss(1,2))
            %warning('The provided matrix is not skew symmetric.')
            %print(ss)
        end

        vec = [ss(3,2); ss(1,3); ss(2,1)];
end

if isa(ss,'sym')
    vec = simplify(vec);
end

end

== matlab function controller_v12/Adaptive Controller/attitude and thrust MPC controller/RTMPC Trajectory Tracking ==
  data: time input; r input; Rd output; r_dot input; r_dotdot input; R input size=9; Omega input; rd input; rd_d input; rd_dd input; rd_ddd input; rd_dddd input; att_cmd input; int_e input; ctr parameter; rbt parameter; Omegad output; cmd_B_acc_z output size=1; mdl parameter; alt_e output; rd_rtmpc output; new_att_cmd output
function [Rd, Omegad, cmd_B_acc_z, alt_e, rd_rtmpc, new_att_cmd]   = fcn(time, r, r_dot, r_dotdot, R, Omega, rd,rd_d,rd_dd,rd_ddd,rd_dddd, att_cmd, int_e, ctr, rbt, mdl)
    %#codegen
    % r: curr pos
    % r_dot: curr vel
    % R: current attitude
    % Omega: current body rates
    % rd : des pos
    % rd_d: des vel
    cmd_B_acc_z = 0;
    %% Out: 
    % cmd_B_thrust_z is thrust force on z axis in body (B) frame [N]
    
    % Ensure signals have expected shape
    R11 = R(1);
    R12 = R(2);
    R13 = R(3);
    R21 = R(4);
    R22 = R(5);
    R23 = R(6);
    R31 = R(7);
    R32 = R(8);
    R33 = R(9);
    R1 = [R11; R21; R31];     % unit (column) vector
    R2 = [R12; R22; R32];
    R3 = [R13; R23; R33];
    R = [R1, R2, R3];

    r = r(:);           % position
    r_dot = r_dot(:);   % velocity 

    rd = rd(:);         % desired position
    rd_d = rd_d(:);     % desired velocity

    new_att_cmd = zeros(2,1);
    Omegad = [0.0; 0.0; 0.0];
    
    % Compute current attitude as euler angles (:( )
    B_ypr = rotm2eul(R);
    B_est_roll = B_ypr(3);
    B_est_pitch = B_ypr(2);
    B_est_yaw = B_ypr(1);

    % Conver attitude in yaw-invariant frame. 
    B_R_yaw_I = get_B_R_yaw_I(B_est_yaw);
    I_rp = B_R_yaw_I'*[B_est_roll; B_est_pitch];

    % Generate reference % (currently only circle is supported)
    x_ref = traj_planner(time, ctr.rtmpc.ref_len, ctr.rtmpc.traj, ctr);

    % Set current state
    x = [r - ctr.rtmpc.r_origin; r_dot; I_rp(1); I_rp(2);];

    if ctr.mode == 0
        % NN RTMPC controller

        % Apply state and reference scaling
        x = [x; att_cmd(1); att_cmd(2)];
        x_scaled = ctr.rtmpc.in_scaling.*x;
        x_ref_scaled = repmat(ctr.rtmpc.in_scaling(1:6), ctr.rtmpc.ref_len, 1).*x_ref;
        
        x_in = [x_scaled; x_ref_scaled];
        x_in = x_in(:); % column vector

        % 10.0 and 12.0 are some scalings applied to the NN to
        % ensure that its input/ouput is in [-1, 1]. 
        % For the rtmpc expert we do not have this care -- but we scale
        % things to ensure that input/outpurs are not too large numbers (e.g., <+-100)
        u_next = 10.0*rtmpcnn(x_in/10.0, ctr.rtmpc.nnparam);

        % Apply rtmpc scaling: 
        u_next = u_next.*ctr.rtmpc.out_scaling;

        % integrated new att cmd
        new_att_cmd = zeros(2,1);
        new_att_cmd(:, 1) = mdl.T*u_next(1:2) + att_cmd;

        % Approach 2: rotate in B after.
        Iy_rp_des_dot = [u_next(1); u_next(2)];
        Iy_rp_des = [new_att_cmd(1); new_att_cmd(2)];
        % compute angular velocity in yaw-aligned frame
        Iy_ypr_des = [0.0; Iy_rp_des(2); Iy_rp_des(1)];
        Iy_ypr_des_dot = [0.0; Iy_rp_des_dot(2); Iy_rp_des_dot(1)];
        Iy_Omegad = get_body_ang_vel(Iy_ypr_des, Iy_ypr_des_dot);
        B_R_yaw_I = get_B_R_yaw_I(B_est_yaw);
        B_Omegad_12 = B_R_yaw_I*Iy_Omegad(1:2);
        Omegad = [B_Omegad_12(1); B_Omegad_12(2); 0.0];
        u_next(1:2) = new_att_cmd;

    elseif ctr.mode == 1
        
        % Set reference 
        %x_ref = [rd; rd_d; 0.0; 0.0]; % no attitude feed-forward at the moment. 
        %mpc.set_reference_trajectory(x_ref);
    
        % Compute new linearized commands
        x = [r; r_dot; I_rp(1); I_rp(2)];

        x_scaled = x.*ctr.lqrv2.in_scaling;
        x_ref_scaled = [x_ref(1:6); 0.0; 0.0;].*ctr.lqrv2.in_scaling;
        u_next = -ctr.lqrv2.K*(x_scaled - x_ref_scaled);
        u_next = u_next.*ctr.lqrv2.out_scaling;
        Omegad = zeros(3, 1);

    elseif ctr.mode == 2
        x = [x; att_cmd(1); att_cmd(2)];
        ctr.lqr.in_scaling = [10; 10; 10; 10; 10; 10; 1; 1; 1; 1];
        x_scaled = x.*ctr.lqr.in_scaling;
        x_ref_scaled = [x_ref(1:6); 0.0; 0.0; 0.0; 0.0;].*ctr.lqr.in_scaling;
        u_next = -ctr.lqr.K*(x_scaled - x_ref_scaled);
        u_next = u_next.*ctr.lqr.out_scaling;

        % integrated new att cmd
        new_att_cmd = zeros(2,1);
        new_att_cmd(:, 1) = mdl.T*u_next(1:2,1) + att_cmd;

        % Approach 1: rotate in B first.
%         I_rp_des_dot = [u_next(1); u_next(2)];
%         B_R_yaw_I = get_B_R_yaw_I(B_est_yaw);
%         B_rp_des_dot = B_R_yaw_I*I_rp_des_dot;
%         B_ypr_des = [B_ypr(1); new_att_cmd(2); new_att_cmd(1)];
%         B_ypr_des_dot = [0.0; B_rp_des_dot(2); B_rp_des_dot(1)];
%         %Omegad = [B_ypr_des_dot(3); B_ypr_des_dot(2); B_ypr_des_dot(1)];
%         Omegad = get_body_ang_vel(B_ypr_des, B_ypr_des_dot);
%         u_next(1:2) = new_att_cmd;

%         % Approach 2: rotate in B after.
        Iy_rp_des_dot = [u_next(1); u_next(2)];
        Iy_rp_des = [new_att_cmd(1); new_att_cmd(2)];
        % compute angular velocity in yaw-aligned frame
        Iy_ypr_des = [0.0; Iy_rp_des(2); Iy_rp_des(1)];
        Iy_ypr_des_dot = [0.0; Iy_rp_des_dot(2); Iy_rp_des_dot(1)];
        Iy_Omegad = get_body_ang_vel(Iy_ypr_des, Iy_ypr_des_dot);
        B_R_yaw_I = get_B_R_yaw_I(B_est_yaw);
        B_Omegad_12 = B_R_yaw_I*Iy_Omegad(1:2);
        Omegad = [B_Omegad_12(1); B_Omegad_12(2); 0.0];
        u_next(1:2) = new_att_cmd;

    else
        disp("ctr.mode not recognized. ")
        u_next= zeros(3, 1);
    end

    rd_rtmpc = x_ref(1:6);
    rd_rtmpc(1:3) = rd_rtmpc(1:3) + ctr.rtmpc.r_origin;
    
    delta_cmd_I_roll =  u_next(1);
    delta_cmd_I_pitch = u_next(2);
    delta_cmd_I_acc_z = u_next(3);
    
    % Compensate thrust
    cmd_B_thrust = compensate_thrust(delta_cmd_I_acc_z, B_ypr, rbt.m, mdl.g);
    cmd_B_thrust_z = cmd_B_thrust(3);
    cmd_B_acc_z = cmd_B_thrust_z/rbt.m;
   
    % apply saturation
    cmd_B_acc_z = max(min(cmd_B_acc_z, mdl.g+2.0), mdl.g-1.0);
    
    % De-rotate attitude commands in body frame
    cmd_I_rp = [delta_cmd_I_roll; delta_cmd_I_pitch];
    B_R_yaw_I = get_B_R_yaw_I(B_est_yaw);
    cmd_B_rp = B_R_yaw_I*cmd_I_rp;

    % Compensate attitude
    if ctr.rtmpc.compensate_attitude
        [cmd_B_roll, cmd_B_pitch] = compensate_attitude(cmd_B_thrust, cmd_B_rp(1), cmd_B_rp(2), rbt.m, mdl.g);
    else
        cmd_B_roll = cmd_B_rp(1);
        cmd_B_pitch = cmd_B_rp(2);
    end
    cmd_B_roll = max(min(cmd_B_roll, ctr.rtmpc.lim.att), -ctr.rtmpc.lim.att);
    cmd_B_pitch = max(min(cmd_B_pitch, ctr.rtmpc.lim.att), -ctr.rtmpc.lim.att);
    cmd_B_yaw = B_est_yaw;

    % Desired angular velocity
    % Omegad = [0.0, 0.0, 0.0]; % TODO
   

    % Altitude error
    alt_e = r(3) - rd(3); 

    freq = 0.25*time;
    %cmd_B_roll = pi/6*square(time*freq);
    %cmd_B_pitch = pi/6*square(time*freq - pi/2);

    %cmd_B_roll = 0.0;
    %cmd_B_pitch = 0.0;
    %cmd_B_yaw = pi/2;
    
    % Desired attitude from RTMPC as rotation matrix
    Rd_tmp = eul2rotm([cmd_B_yaw, cmd_B_pitch, cmd_B_roll]); % intrinsic, zyx


    % Eq 15 of Lee2010: treat I_T from mpc as (-kxex -kvev - mge3 + mxdd):
    %e3 = [0; 0; 1];
    %cmd_B_acc_z = (Rd_tmp*[0; 0; cmd_B_acc_z])'*R*e3;

%     %%% TODO: Andrea: remove
%     % Try flip
%     speedf = 5.0;
%     if (time > 1.0) && (time < (1.0 + 1.0/speedf))
%         Rd_tmp = axang2rotm([-1, 0, 0, speedf*2.0*pi*(1.0 - time)]);
%         Omegad = [speedf*2.0*pi, 0.0, 0.0];
%     end
%     %%% 

    % Generate output. 
    Rd_tmp = Rd_tmp'; % this is needed to respect existing convention that rot. matrices are passed
          % around as vectors, created by concatenating the rows of the
          % matrix (and Rd(:) will created a vector by concatentatig the columns of Rd)
    Rd = Rd_tmp(:);
end

function [B_thrust] = compensate_thrust(cmd_B_acc_z, B_ypr, mass, g)
    B_thrust_z = mass * (cmd_B_acc_z+g)/cos(B_ypr(3))/cos(B_ypr(2));
    B_thrust = [0.0; 0.0; B_thrust_z];
end

function [B_roll, B_pitch] = compensate_attitude(B_thrust, lin_B_roll, lin_B_pitch, mass, g)
    B_acc_z = (B_thrust(3))/mass;
    B_roll = lin_B_roll*(g/B_acc_z);
    B_pitch = lin_B_pitch*(g/B_acc_z);
end

function [R] = get_B_R_yaw_I(yaw)
    R = [cos(yaw), sin(yaw); -sin(yaw), cos(yaw)];
end

function [B_omega] = get_body_ang_vel(B_ypr, B_ypr_dot)
% https://www.astro.rug.nl/software/kapteyn-beta/_downloads/attitude.pdf
sy = sin(B_ypr(1));
cy = cos(B_ypr(1));
sp = sin(B_ypr(2));
cp = cos(B_ypr(2));
E_zyx = [[0; 0; 1], [-sy; cy; 0.0], [cy*cp; sy*cp; -sp]];
B_omega = E_zyx*B_ypr_dot;

end

== matlab function controller_v12/Adaptive Controller/observer/ICRA'23/Rotaion/Rotation Matrix1 ==
  data: R input; Rdot input; w output
function w  = fcn(R,Rdot)
%#codegen
w = zeros(3,1);
w(1) = R(3)*Rdot(2) + R(6)*Rdot(5) + R(9)*Rdot(8);
w(2) = R(1)*Rdot(3) + R(4)*Rdot(6) + R(7)*Rdot(9);
w(3) = R(2)*Rdot(1) + R(5)*Rdot(4) + R(8)*Rdot(7);

== matlab function controller_v12/Adaptive Controller/attitude and thrust MPC controller/Rotm2rpy ==
  data: R input; rpy output size=3
function rpy  = fcn(R)
    R = get_rotation_matrix(R);
    ypr = rotm2eul(R); 
    rpy = squeeze([ypr(3); ypr(2); ypr(1)]);

end

function R = get_rotation_matrix(R)
    R11 = R(1);
    R12 = R(2);
    R13 = R(3);
    R21 = R(4);
    R22 = R(5);
    R23 = R(6);
    R31 = R(7);
    R32 = R(8);
    R33 = R(9);
    R1 = [R11; R21; R31];     % unit (column) vector
    R2 = [R12; R22; R32];
    R3 = [R13; R23; R33];
    R = [R1, R2, R3];
end

== matlab function controller_v12/Adaptive Controller/attitude and thrust MPC controller/Rotm2rpy1 ==
  data: R input; rpy output size=3
function rpy   = fcn(R)
    R = get_rotation_matrix(R);
    ypr = rotm2eul(R); 
    rpy = [ypr(3); ypr(2); ypr(1)];
end

function R = get_rotation_matrix(R)
    R11 = R(1);
    R12 = R(2);
    R13 = R(3);
    R21 = R(4);
    R22 = R(5);
    R23 = R(6);
    R31 = R(7);
    R32 = R(8);
    R33 = R(9);
    R1 = [R11; R21; R31];     % unit (column) vector
    R2 = [R12; R22; R32];
    R3 = [R13; R23; R33];
    R = [R1, R2, R3];
end
